simulink model "Overcurrent"  (R2024a)
settings: Solver=VariableStepAuto  StartTime=0.0  StopTime=10.0  RelTol=1e-3
libraries: spsRMSLib x3, simulink_extras x3
settings Model: Creator=MEET  LastModifiedBy=MEET

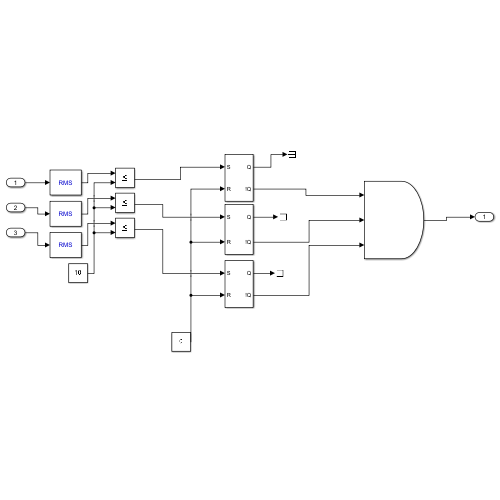
[thumbnail: Simulink's stored preview of the top-level diagram]
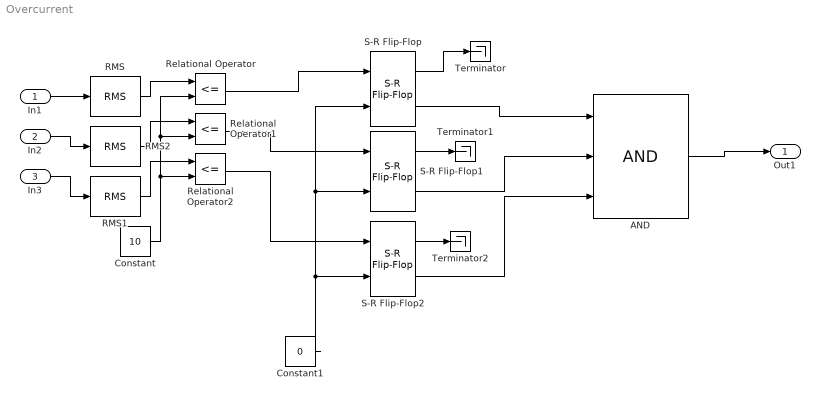
== system Overcurrent ==
  In1 : Inport
  In2 : Inport  Port=2
  In3 : Inport  Port=3
  AND : Logic  Inputs=3  IconShape=distinctive  AllPortsSameDT=off  OutDataTypeStr=boolean
  Constant : Constant  Value=10
  Constant1 : Constant  Value=0
  RMS : spsRMSLib/RMS  TrueRMS=on  Freq=50  RMSInit=0  Ts=0.001
  RMS1 : spsRMSLib/RMS  TrueRMS=on  Freq=50  RMSInit=0  Ts=0.001
  RMS2 : spsRMSLib/RMS  TrueRMS=on  Freq=50  RMSInit=0  Ts=0.001
  Relational Operator : RelationalOperator  Operator=<=  OutDataTypeStr=boolean  RndMeth=Simplest  InputSameDT=off
  Relational Operator1 : RelationalOperator  Operator=<=  OutDataTypeStr=boolean  RndMeth=Simplest  InputSameDT=off
  Relational Operator2 : RelationalOperator  Operator=<=  OutDataTypeStr=boolean  RndMeth=Simplest  InputSameDT=off
  S-R Flip-Flop : simulink_extras/Flip Flops/S-R Flip-Flop  initial_condition=0
  S-R Flip-Flop1 : simulink_extras/Flip Flops/S-R Flip-Flop  initial_condition=0
  S-R Flip-Flop2 : simulink_extras/Flip Flops/S-R Flip-Flop  initial_condition=0
  Terminator : Terminator
  Terminator1 : Terminator
  Terminator2 : Terminator
  Out1 : Outport
  wires:
  Constant/1 -> Relational Operator2/2, Relational Operator1/2, Relational Operator/2
  Constant1/1 -> S-R Flip-Flop2/2, S-R Flip-Flop1/2, S-R Flip-Flop/2
  Relational Operator/1 -> S-R Flip-Flop/1
  Relational Operator1/1 -> S-R Flip-Flop1/1
  Relational Operator2/1 -> S-R Flip-Flop2/1
  AND/1 -> Out1/1
  In1/1 -> RMS/1
  In2/1 -> RMS2/1
  In3/1 -> RMS1/1
  RMS/1 -> Relational Operator/1
  RMS2/1 -> Relational Operator1/1
  RMS1/1 -> Relational Operator2/1
  S-R Flip-Flop/2 -> AND/1
  S-R Flip-Flop1/2 -> AND/2
  S-R Flip-Flop2/2 -> AND/3
  S-R Flip-Flop2/1 -> Terminator2/1
  S-R Flip-Flop1/1 -> Terminator1/1
  S-R Flip-Flop/1 -> Terminator/1
